simulink model "IE474_O1_Task2_simulink_X"  (Simulink 9.3)
settings: Solver=VariableStepAuto  StartTime=0.0  StopTime=10.0  RelTol=1e-3
values from neighbouring files (symbols this model uses):
  a = a_vec(ii)    [driver.m]
  b = b_vec(ii)    [driver.m]
  K = K_vec(ii)    [driver.m]
settings Model: Creator=Radium  LastModifiedBy=Radium
settings DataIOCC: FinalStateName=xfinal  SignalLoggingSaveFormat=Dataset
settings OptimizationCC: LifeSpan=auto
settings DebuggingCC: UnderspecifiedInitializationDetection=Simplified  MergeDetectMultiDrivingBlocksExec=error  FcnCallInpInsideContextMsg=error  SFUnexpectedBacktrackingDiag=error  SFNoUnconditionalDefaultTransitionDiag=error  SFExecutionAtInitializationDiag=warning  ArithmeticOperatorsInVariantConditions=error
settings HardwareCC: ProdBitPerPointer=64  ProdBitPerSizeT=64  ProdBitPerPtrDiffT=64  ProdLargestAtomicFloat=Float  ProdIntDivRoundTo=Zero  ProdEndianess=LittleEndian  ProdWordSize=64  ProdHWDeviceType=Intel->x86-64 (Windows64)
settings ModelReferenceCC: PropagateSignalLabelsOutOfModel=on
settings SFSimCC: SimUseLocalCustomCode=on
settings RTWCC: RTWUseLocalCustomCode=on
settings CodeAppCC: StateflowObjectComments=off
settings GRTTargetCC: TargetLangStandard=C99 (ISO)  CombineOutputUpdateFcns=on  GRTInterface=off
settings ConfigComp: CovMetricSettings=dwe  CovHtmlReporting=off  CovSaveCumulativeToWorkspaceVar=off  CovSaveSingleToWorkspaceVar=off  CovExternalEMLEnable=on

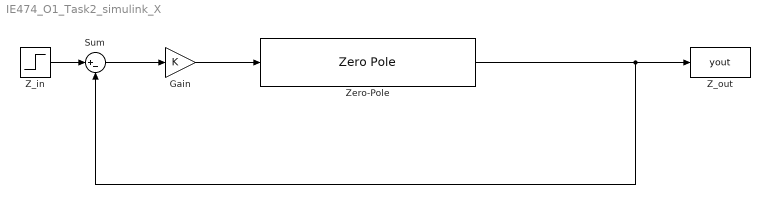
== system IE474_O1_Task2_simulink_X ==
  Gain : Gain  Gain=K
  Sum : Sum  Inputs=|+-
  Z_in : Step  After=0.1  SampleTime=0
  Z_out : ToWorkspace  VariableName=yout  SampleTime=-1
      settings: Save2DSignal=2-D array (concatenate along first dimension)
  Zero-Pole : ZeroPole  Zeros=[-a -b]  Poles=[0 62.61 -62.61]  Gain=[7570]
  wires:
  Zero-Pole/1 -> Sum/2, Z_out/1
  Sum/1 -> Gain/1
  Gain/1 -> Zero-Pole/1
  Z_in/1 -> Sum/1
